simulink model "my_macro2025b"  (R2025b)
settings: Solver=VariableStepAuto
values from neighbouring files (symbols this model uses):
  K = lqr(A, B, Qr, Rr)    [Home1.m]    (also in IP_MACRO.m; testes_30_03.m)
undefined symbols (not defined in the file or in its folder): data
settings Model: Creator=sofia  LastModifiedBy=sofia
settings DataIOCC: ReturnWorkspaceOutputs=off

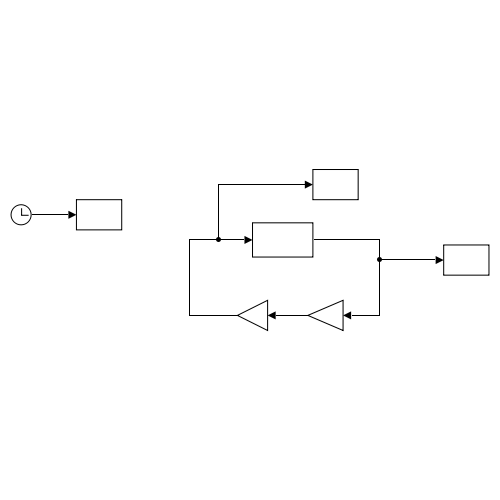
[thumbnail: Simulink's stored preview of the top-level diagram]
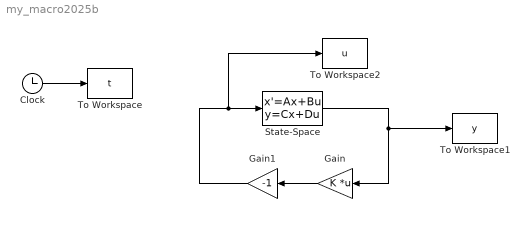
== system my_macro2025b ==
  Clock : Clock
  Gain : Gain  Gain=K  Multiplication=Matrix(K*u)
  Gain1 : Gain  Gain=-1
  State-Space : StateSpace  A=data.A  B=data.B  C=eye(5)  D=[0 0 0 0 0]'  InitialCondition=1  ContinuousStateAttributes={'x1','x2','x3','x4','x5'}
  To Workspace : ToWorkspace  VariableName=t  SaveFormat=Timeseries  SampleTime=-1
  To Workspace1 : ToWorkspace  VariableName=y  SampleTime=-1
      settings: Save2DSignal=2-D array (concatenate along first dimension)
  To Workspace2 : ToWorkspace  VariableName=u  SampleTime=-1
      settings: Save2DSignal=2-D array (concatenate along first dimension)
  wires:
  Gain1/1 -> To Workspace2/1, State-Space/1
  State-Space/1 -> Gain/1, To Workspace1/1
  Gain/1 -> Gain1/1
  Clock/1 -> To Workspace/1
